simulink model "UAM_Flight_control"  (R2024b)
settings: Solver=FixedStepAuto  StartTime=0.0  StopTime=inf  RelTol=1e-3  EnableMultiTasking=on
undefined symbols (not defined in the file): CityMission, control, controlParams, ControlSampleTime, Cruise_a, DiscIntNeverNeededParam, Earth, FixedWingMission, flightState, FSState, FWControlParams, FWTrimSpeed, HoverMission, params, position, R_WAYPOINTTRANSITION, TransitionMission, uavParam, Vt, w_trim, WGS84, zGround
libraries: slpidlib x56, simulink x35, uavalgslib x8, robotcorelib x2, simulink_extras x2, mspfiltlib x1, aerolibtransform2 x1
(part 3 of 12)

== system UAM_Flight_control/GNC/Guidance/Auto ==
  note: Ground : 해발고도 기준, 착륙 지점 고도
  Pose : Inport
  Mission : Inport  Port=2  OutDataTypeStr=Bus: UAVPathManagerBus
  isModeDone : Inport  Port=3
  LandingStates : Inport  Port=4
  States : Inport  Port=5
  Ground : Inport  Port=6
  Action Port : ActionPort  ActionPortLabel=case [ Auto ]:
  Bus Creator : BusCreator  Inputs=6  OutDataTypeStr=Bus: GNCplan
  Bus Creator1 : BusCreator  Inputs=3  OutDataTypeStr=Bus: UAVPathManagerBus  NonVirtualBus=on
  Bus Selector : BusSelector  OutputSignals=mode
  Bus Selector1 : BusSelector  OutputSignals=target
  Compare To Constant : simulink/Logic and Bit Operations/Compare To Constant  relop===  const=1  OutDataTypeStr=boolean
  Compare To Constant1 : simulink/Logic and Bit Operations/Compare To Constant  relop=>=  const=3.0  OutDataTypeStr=boolean
  Constant : Constant  Value=0  OutDataTypeStr=uint8
  Constant1 : Constant  Value=[0,0,0]  OutDataTypeStr=double
  Constant2 : Constant  OutDataTypeStr=uint8
  Constant3 : Constant  Value=[0;0;0;0]
  Goto : Goto  Commented=on  GotoTag=landingState
  IC : InitialCondition
  Logical Operator : Logic  Operator=OR  Inputs=1  AllPortsSameDT=off  OutDataTypeStr=boolean
  Path Manager : uavalgslib/Path Manager  UAVType=multirotor  LoiterRadius=25  dataType=double  inputBusName='UAVPathManagerBus'  SimulateUsing=Code generation
  Reshape : Reshape  OutputDimensionality=Customize  OutputDimensions=[3 1]
  Selector : Selector  InputPortWidth=2  IndexOptions=Index vector (dialog)  Indices=1  OutputSizes=1
  Selector1 : Selector  InputPortWidth=2  IndexOptions=Index vector (dialog)  Indices=2  OutputSizes=1
  Switch : Switch  Criteria=u2 > Threshold  SaturateOnIntegerOverflow=off  InputSameDT=off
  GNCPlan : Outport  OutDataTypeStr=Bus: GNCplan
  wires:
  IC/1 -> Bus Creator/1  "mode"
  Ground/1 -> Bus Creator/6  "ground"
  Selector1/1 -> Bus Creator/3  "FromWP"
  States/1 -> Bus Selector1/1, Bus Creator/5  "states"
  Bus Creator/1 -> GNCPlan/1
  Selector/1 -> Bus Selector/1, Switch/3  "ToWP"
  Path Manager/1 -> Selector/1, Selector1/1
  Constant/1 -> Path Manager/4
  Constant1/1 -> Path Manager/5
  Pose/1 -> Bus Creator/4, Path Manager/1  "pose"
  LandingStates/1 -> Goto/1
  Compare To Constant/1 -> Path Manager/3
  isModeDone/1 -> Compare To Constant/1
  Bus Selector/1 -> IC/1  "<mode>"
  Mission/1 -> Path Manager/2
  Bus Selector1/1 -> Reshape/1, Compare To Constant1/1  "<target>"
  Compare To Constant1/1 -> Logical Operator/1
  Logical Operator/1 -> Switch/2
  Switch/1 -> Bus Creator/2  "ToWP"
  Constant2/1 -> Bus Creator1/1  "mode"
  Constant3/1 -> Bus Creator1/3  "params"
  Reshape/1 -> Bus Creator1/2  "position"
  Bus Creator1/1 -> Switch/1

== system UAM_Flight_control/GNC/Guidance/Emergency ==
  pose : Inport
  states : Inport  Port=2
  ground : Inport  Port=3
  Action Port : ActionPort  ActionPortLabel=case [ Emergecny ]:
  Bus Creator : BusCreator  Inputs=6  OutDataTypeStr=Bus: GNCplan
  Constant1 : Constant  Value=struct('mode', uint8(0), 'position', zeros(3,1), 'params', zeros(4,1))  OutDataTypeStr=Bus: UAVPathManagerBus
  Constant2 : Constant  Value=struct('mode', uint8(0), 'position', zeros(3,1), 'params', zeros(4,1))  OutDataTypeStr=Bus: UAVPathManagerBus
  Constant3 : Constant  Value=0  OutDataTypeStr=uint8
  GNCPlan : Outport  OutDataTypeStr=Bus: GNCplan
  wires:
  pose/1 -> Bus Creator/4  "pose"
  Bus Creator/1 -> GNCPlan/1
  Constant1/1 -> Bus Creator/2  "ToWP"
  Constant2/1 -> Bus Creator/3  "FromWP"
  ground/1 -> Bus Creator/6  "ground"
  states/1 -> Bus Creator/5  "states"
  Constant3/1 -> Bus Creator/1  "mode"

== system UAM_Flight_control/GNC/Guidance/Switch Case Action Subsystem ==
  pose : Inport
  states : Inport  Port=2
  ground : Inport  Port=3
  Action Port : ActionPort  ActionPortLabel=case [ Manual ]:
  Bus Creator : BusCreator  Inputs=6  OutDataTypeStr=Bus: GNCplan
  Constant1 : Constant  Value=struct('mode', uint8(0), 'position', zeros(3,1), 'params', zeros(4,1))  OutDataTypeStr=Bus: UAVPathManagerBus
  Constant2 : Constant  Value=struct('mode', uint8(0), 'position', zeros(3,1), 'params', zeros(4,1))  OutDataTypeStr=Bus: UAVPathManagerBus
  Constant3 : Constant  Value=0  OutDataTypeStr=uint8
  GNCPlan : Outport  OutDataTypeStr=Bus: GNCplan
  wires:
  Bus Creator/1 -> GNCPlan/1
  Constant3/1 -> Bus Creator/1  "mode"
  Constant2/1 -> Bus Creator/3  "FromWP"
  Constant1/1 -> Bus Creator/2  "ToWP"
  pose/1 -> Bus Creator/4  "pose"
  states/1 -> Bus Creator/5  "states"
  ground/1 -> Bus Creator/6  "ground"

== system UAM_Flight_control/GNC/Guidance/UAM POS ==
  UAMStates : Inport  OutDataTypeStr=Bus: StateBus
  Bus Creator : BusCreator  Inputs=5
  Bus Selector : BusSelector  OutputSignals=Xe,Ve
  Demux : Demux  Outputs=3
  Display : Display
  Selector : Selector  InputPortWidth=3  IndexOptions=Index vector (dialog)  Indices=[1]  OutputSizes=1
  Selector1 : Selector  InputPortWidth=3  IndexOptions=Index vector (dialog)  Indices=[2]  OutputSizes=1
  POS : Outport
  wires:
  UAMStates/1 -> Bus Selector/1
  Bus Selector/1 -> Demux/1  "<Xe>"
  Demux/1 -> Bus Creator/1  "x"
  Demux/2 -> Bus Creator/2  "y"
  Demux/3 -> Bus Creator/3  "z"
  Bus Selector/2 -> Selector/1, Selector1/1  "<Ve>"
  Selector/1 -> Bus Creator/4  "vx"
  Selector1/1 -> Bus Creator/5  "vy"
  Bus Creator/1 -> Display/1, POS/1

== system UAM_Flight_control/GNC/Guidance/UAM States ==
  UAMStates : Inport
  Bus Creator : BusCreator  Inputs=8
  Bus Selector : BusSelector  OutputSignals=Euler,pqr,Ve,Xe,course,RotorParameters,RC,target
  States : Outport
  wires:
  UAMStates/1 -> Bus Selector/1
  Bus Creator/1 -> States/1
  Bus Selector/1 -> Bus Creator/1  "<Euler>"
  Bus Selector/2 -> Bus Creator/2  "<pqr>"
  Bus Selector/3 -> Bus Creator/3  "<Ve>"
  Bus Selector/5 -> Bus Creator/5  "<course>"
  Bus Selector/4 -> Bus Creator/4  "<Xe>"
  Bus Selector/6 -> Bus Creator/6  "<RotorParameters>"
  Bus Selector/7 -> Bus Creator/7  "<RC>"
  Bus Selector/8 -> Bus Creator/8  "<target>"

== system UAM_Flight_control/GNC/Navigation/LLA2Local ==
  LLA : Inport
  ve : Inport  Port=2
  Enabled Subsystem : Subsystem  Commented=on  TreatAsAtomicUnit=on
  MATLAB Function : MATLAB Function  TreatAsAtomicUnit=on
  Xe : Outport
  wires:
  LLA/1 -> MATLAB Function/1(LLA)
  ve/1 -> MATLAB Function/2(arming)
  MATLAB Function/1(Xe) -> Xe/1

== system UAM_Flight_control/Sensor/Subsystem1/Subsystem ==
  Inport : Inport
  Gain2 : Gain  Gain=0.5
  Gyro_bias : Constant  Value=[-0.000114; -0.000246; -0.001536]
  MATLAB Function1 : MATLAB Function  TreatAsAtomicUnit=on
  MATLAB Function2 : MATLAB Function  TreatAsAtomicUnit=on
  Sum : Sum  Inputs=|+-
  Unit Delay : UnitDelay  InitialCondition=[1;0;0;0]  SampleTime=-1  HasFrameUpgradeWarning=on
  dt : Gain  Gain=0.005
  normalize : MATLAB Function  TreatAsAtomicUnit=on
  qn : Outport
  wires:
  Sum/1 -> Gain2/1
  MATLAB Function2/1(qout) -> normalize/1(q)
  normalize/1(qn) -> qn/1, Unit Delay/1
  Gyro_bias/1 -> Sum/2
  Unit Delay/1 -> MATLAB Function2/1(q)
  Gain2/1 -> dt/1
  Inport/1 -> Sum/1
  dt/1 -> MATLAB Function1/1(theta)
  MATLAB Function1/1(dq) -> MATLAB Function2/2(dq)

== system UAM_Flight_control/Controller/Auto1/Blend Scheduler/BTalpha ==
  States : Inport
  Bus Selector : BusSelector  OutputSignals=airspeed
  Constant : Constant  Value=65
  Gain : Gain  Gain=1/20
  Saturation : Saturate  UpperLimit=1  LowerLimit=0
  Subtract : Sum  Inputs=+-
  alpha : Outport
  wires:
  Constant/1 -> Subtract/1
  Subtract/1 -> Gain/1
  Gain/1 -> Saturation/1
  Saturation/1 -> alpha/1
  States/1 -> Bus Selector/1
  Bus Selector/1 -> Subtract/2  "<airspeed>"

== system UAM_Flight_control/Controller/Auto1/Blend Scheduler/FTalpha ==
  States : Inport
  1-a : Sum  Inputs=+-
  Bus Selector : BusSelector  OutputSignals=airspeed
  Constant3 : Constant  Value=35
  Constant5 : Constant  Value=Cruise_a
  Gain3 : Gain  Gain=1/10
  Saturation1 : Saturate  UpperLimit=10  LowerLimit=0
  Sum2 : Sum  Inputs=|+-
  alpha : Outport
  wires:
  1-a/1 -> alpha/1
  Bus Selector/1 -> Sum2/1  "<airspeed>"
  Gain3/1 -> 1-a/2
  Sum2/1 -> Saturation1/1
  Saturation1/1 -> Gain3/1
  Constant3/1 -> Sum2/2
  States/1 -> Bus Selector/1
  Constant5/1 -> 1-a/1

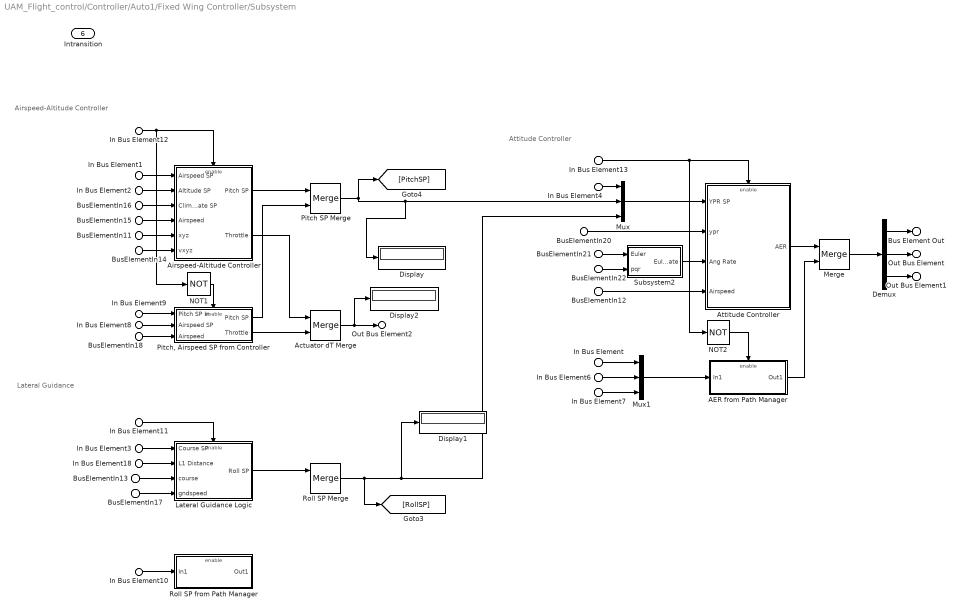
== system UAM_Flight_control/Controller/Auto1/Fixed Wing Controller/Subsystem ==
  note: Airspeed-Altitude Controller
  note: Lateral Guidance
  note: Attitude Controller
  BusElementIn11 : Inport  PortName=States  Element=Xe
  BusElementIn12 : Inport  PortName=States  Element=airspeed
  BusElementIn15 : Inport  PortName=States  Element=airspeed
  BusElementIn18 : Inport  PortName=States  Element=airspeed
  BusElementIn13 : Inport  PortName=States  Element=course
  BusElementIn16 : Inport  PortName=States  Element=course
  BusElementIn14 : Inport  PortName=States  Element=Ve_ground
  BusElementIn17 : Inport  PortName=States  Element=gndspeed
  BusElementIn20 : Inport  PortName=States  Element=YPR
  BusElementIn21 : Inport  PortName=States  Element=Euler
  BusElementIn22 : Inport  PortName=States  Element=pqr
  In Bus Element11 : Inport  Port=2  PortName=Control Mode  Element=lateralGuidance
  In Bus Element12 : Inport  Port=2  PortName=Control Mode  Element=airspeedAltitude
  In Bus Element13 : Inport  Port=2  PortName=Control Mode  Element=attitude
  In Bus Element1 : Inport  Port=3  PortName=AAC SP  Element=airspeed
  In Bus Element2 : Inport  Port=3  PortName=AAC SP  Element=altitude
  In Bus Element18 : Inport  Port=3  PortName=AAC SP  Element=L1
  In Bus Element3 : Inport  Port=3  PortName=AAC SP  Element=course
  In Bus Element4 : Inport  Port=4  PortName=FixedWingSP  Element=yaw
  In Bus Element9 : Inport  Port=4  PortName=FixedWingSP  Element=pitch
  In Bus Element10 : Inport  Port=4  PortName=FixedWingSP  Element=roll
  In Bus Element8 : Inport  Port=4  PortName=FixedWingSP  Element=airspeed
  In Bus Element : Inport  Port=5  PortName=AERT  Element=aileron
  In Bus Element6 : Inport  Port=5  PortName=AERT  Element=elevator
  In Bus Element7 : Inport  Port=5  PortName=AERT  Element=rudder
  Intransition : Inport  Port=6
  AER from Path Manager : Subsystem  TreatAsAtomicUnit=on
  Actuator dT Merge : Merge
  Airspeed-Altitude Controller : Subsystem
  Attitude Controller : Subsystem
  Demux : Demux  Outputs=3
  Display : Display
  Display1 : Display
  Display2 : Display
  Lateral Guidance Logic : Subsystem
  Merge : Merge
  Mux : Mux  Inputs=3
  Mux1 : Mux  Inputs=3
  NOT1 : Logic  Operator=NOT  IconShape=distinctive  AllPortsSameDT=off  OutDataTypeStr=boolean
  NOT2 : Logic  Operator=NOT  IconShape=distinctive  AllPortsSameDT=off  OutDataTypeStr=boolean
  Pitch SP Merge : Merge
  "Pitch, Airspeed SP from Controller" : Subsystem  TreatAsAtomicUnit=on
  Roll SP Merge : Merge
  Roll SP from Path Manager : Subsystem  TreatAsAtomicUnit=on
  Subsystem2 : Subsystem
  Bus Element Out : Outport  PortName=Actuator  Element=dA
  Out Bus Element : Outport  PortName=Actuator  Element=dE
  Out Bus Element1 : Outport  PortName=Actuator  Element=dR
  Out Bus Element2 : Outport  PortName=Actuator  Element=dT
  wires:
  In Bus Element4/1 -> Mux/1
  Roll SP Merge/1 -> [RollSP], Display1/1, Mux/3
  BusElementIn18/1 -> "Pitch, Airspeed SP from Controller"/3(Airspeed)
  In Bus Element12/1 -> Airspeed-Altitude Controller/Enable, NOT1/1
  In Bus Element3/1 -> Lateral Guidance Logic/1(Course SP)
  Mux1/1 -> AER from Path Manager/1(In1)
  In Bus Element11/1 -> Lateral Guidance Logic/Enable
  Lateral Guidance Logic/1(Roll SP) -> Roll SP Merge/1
  In Bus Element7/1 -> Mux1/3
  Demux/2 -> Out Bus Element/1
  Demux/1 -> Bus Element Out/1
  In Bus Element9/1 -> "Pitch, Airspeed SP from Controller"/1(Pitch SP In)
  Merge/1 -> Demux/1
  In Bus Element18/1 -> Lateral Guidance Logic/2(L1 Distance)
  In Bus Element13/1 -> NOT2/1, Attitude Controller/Enable
  "Pitch, Airspeed SP from Controller"/1(Pitch SP) -> Pitch SP Merge/2
  BusElementIn14/1 -> Airspeed-Altitude Controller/6(vxyz)
  Pitch SP Merge/1 -> Display/1, Mux/2, [PitchSP]
  BusElementIn15/1 -> Airspeed-Altitude Controller/4(Airspeed)
  In Bus Element8/1 -> "Pitch, Airspeed SP from Controller"/2(Airspeed SP)
  BusElementIn13/1 -> Lateral Guidance Logic/3(course)
  Airspeed-Altitude Controller/2(Throttle) -> Actuator dT Merge/1
  BusElementIn16/1 -> Airspeed-Altitude Controller/3(Climb Rate SP)
  In Bus Element1/1 -> Airspeed-Altitude Controller/1(Airspeed SP)
  BusElementIn11/1 -> Airspeed-Altitude Controller/5(xyz)
  BusElementIn12/1 -> Attitude Controller/4(Airspeed)
  In Bus Element2/1 -> Airspeed-Altitude Controller/2(Altitude SP)
  BusElementIn20/1 -> Attitude Controller/2(ypr)
  Mux/1 -> Attitude Controller/1(YPR SP)
  Demux/3 -> Out Bus Element1/1
  BusElementIn21/1 -> Subsystem2/1(Euler)
  Subsystem2/1(Euler Rate) -> Attitude Controller/3(Ang Rate)
  "Pitch, Airspeed SP from Controller"/2(Throttle) -> Actuator dT Merge/2
  Airspeed-Altitude Controller/1(Pitch SP) -> Pitch SP Merge/1
  Attitude Controller/1(AER) -> Merge/1
  AER from Path Manager/1(Out1) -> Merge/2
  In Bus Element/1 -> Mux1/1
  In Bus Element10/1 -> Roll SP from Path Manager/1(In1)
  In Bus Element6/1 -> Mux1/2
  NOT2/1 -> AER from Path Manager/Enable
  BusElementIn22/1 -> Subsystem2/2(pqr)
  Actuator dT Merge/1 -> Display2/1, Out Bus Element2/1
  BusElementIn17/1 -> Lateral Guidance Logic/4(gndspeed)
  NOT1/1 -> "Pitch, Airspeed SP from Controller"/Enable

== system UAM_Flight_control/Controller/Auto1/Multicopter Controller/Attitude & Altitude controller ==
  Ref Attitude : Inport
  States : Inport  Port=2
  Z ref : Inport  Port=3
  InTransition : Inport  Port=4
  CtrlMode : Inport  Port=5
  FlightMode : Inport  Port=6
  Altitude Control : Subsystem
  Bus Selector : BusSelector  OutputSignals=RC
  Compare To Constant : simulink/Logic and Bit Operations/Compare To Constant  relop=>  const=1700  OutDataTypeStr=boolean
  Derivative Gain : Subsystem  VariantControl=AttitudeControl==1
  Selector : Selector  InputPortWidth=10  IndexOptions=Index vector (dialog)  Indices=7  OutputSizes=1
  Roll torque cmd : Outport
  Pitch torque Cmd : Outport  Port=2
  Yaw torque Cmd : Outport  Port=3
  commanded thrust : Outport  Port=4
  wires:
  Altitude Control/1(commanded thrust) -> commanded thrust/1
  Derivative Gain/1(Roll torque cmd) -> Roll torque cmd/1
  InTransition/1 -> Altitude Control/3(InTransition)
  Derivative Gain/2(Pitch torque Cmd) -> Pitch torque Cmd/1
  States/1 -> Derivative Gain/2(States), Bus Selector/1, Altitude Control/1(States)
  Derivative Gain/3(Yaw torque Cmd) -> Yaw torque Cmd/1
  Z ref/1 -> Altitude Control/2(Z ref)
  FlightMode/1 -> Altitude Control/4(FlightMode)
  Ref Attitude/1 -> Derivative Gain/1(Ref Attitude)
  Selector/1 -> Compare To Constant/1
  Bus Selector/1 -> Selector/1  "<RC>"
  Compare To Constant/1 -> Altitude Control/Enable
  CtrlMode/1 -> Derivative Gain/3(CtrlMode), Altitude Control/5(CtrlMode)

== system UAM_Flight_control/Controller/Auto1/Multicopter Controller/Horizontal Position Control ==
  note: Forward Motion is controlled using Tilt.
      | Lateral Motion occurs using roll.
  XRef : Inport
  YRef : Inport  Port=2
  States : Inport  Port=3
  Enable : EnablePort  ShowOutputPort=on
  Signal Conversion : SignalConversion  OverrideOpt=off
  Signal Conversion1 : SignalConversion  OverrideOpt=off
  XY Controller : Subsystem
  Roll Cmd : Outport
  Pitch Cmd : Outport  Port=2
  wires:
  XRef/1 -> XY Controller/1(X_ref)
  YRef/1 -> XY Controller/2(Y_ref)
  States/1 -> XY Controller/3(States)
  XY Controller/1(Forward cmd) -> Signal Conversion/1
  XY Controller/2(Sideward Cmd) -> Signal Conversion1/1
  Signal Conversion/1 -> Pitch Cmd/1
  Signal Conversion1/1 -> Roll Cmd/1
  Enable/1 -> XY Controller/Enable

== system UAM_Flight_control/Controller/Auto1/Multicopter Controller/Organize Inputs ==
  forward command : Inport
  commanded phi torque : Inport  Port=2
  commanded theta torque : Inport  Port=3
  commanded psi torque : Inport  Port=4
  commanded thrust : Inport  Port=5
  Out Bus Element : Outport  PortName=MixerCommands  Element=w_phi
  Out Bus Element1 : Outport  PortName=MixerCommands  Element=w_theta
  Out Bus Element2 : Outport  PortName=MixerCommands  Element=w_psi
  Out Bus Element3 : Outport  PortName=MixerCommands  Element=w_z
  Out Bus Element4 : Outport  PortName=MixerCommands  Element=l_x
  wires:
  forward command/1 -> Out Bus Element4/1
  commanded phi torque/1 -> Out Bus Element/1  "phi"
  commanded theta torque/1 -> Out Bus Element1/1
  commanded psi torque/1 -> Out Bus Element2/1
  commanded thrust/1 -> Out Bus Element3/1

== system UAM_Flight_control/Controller/Auto1/Multicopter Controller/transition controller ==
  Enable : EnablePort
  Constant : Constant  Value=0
  Constant1 : Constant  Value=0
  Rollcmd : Outport
  Pitchcmd : Outport  Port=2
  wires:
  Constant/1 -> Rollcmd/1
  Constant1/1 -> Pitchcmd/1

== system UAM_Flight_control/Controller/Auto1/Scheduler/FixedWingScheduler ==
  note: C opyright 2024 The MathWorks, Inc.
  note: Fixed Wing Control Mixer
  FlightState : Inport
  FixedWingActuators : Inport  Port=2  OutDataTypeStr=Bus: FixedWingCtrlBus
  Merge : Merge  Inputs=4
  Switch Case : SwitchCase  CaseConditions={flightState.Hover, flightState.Transition, flightState.FixedWing,flightState.BackTransition}  ShowDefaultCase=off
  Switch Case Action Subsystem : Subsystem  TreatAsAtomicUnit=on
  Switch Case Action Subsystem1 : Subsystem  TreatAsAtomicUnit=on
  Switch Case Action Subsystem2 : Subsystem  TreatAsAtomicUnit=on
  Switch Case Action Subsystem3 : Subsystem  TreatAsAtomicUnit=on
  ActuatorControls : Outport
  wires:
  FlightState/1 -> Switch Case/1
  FixedWingActuators/1 -> Switch Case Action Subsystem2/1(FixedWingActuators), Switch Case Action Subsystem1/1(FixedWingActuators)
  Switch Case/3 -> Switch Case Action Subsystem2/Action
  Switch Case/2 -> Switch Case Action Subsystem1/Action
  Switch Case Action Subsystem3/1(FixedWingControls) -> Merge/4
  Merge/1 -> ActuatorControls/1
  Switch Case Action Subsystem1/1(FixedWingControls) -> Merge/2
  Switch Case/4 -> Switch Case Action Subsystem3/Action
  Switch Case Action Subsystem/1(FixedWingControls) -> Merge/1
  Switch Case/1 -> Switch Case Action Subsystem/Action
  Switch Case Action Subsystem2/1(FixedWingControls) -> Merge/3

== system UAM_Flight_control/Controller/Auto1/Scheduler/Subsystem ==
  note: C opyright 2024 The MathWorks, Inc.
  note: Multicopter Control Mixer
  FlightState : Inport
  FixedWingActuators : Inport  Port=2
  CtrlMode : Inport  Port=3
  MotorCommands : Inport  Port=4
  Actuator To Voltage : Subsystem
  Merge : Merge  Inputs=4
  Switch Case : SwitchCase  CaseConditions={flightState.Hover, flightState.Transition, flightState.FixedWing,flightState.BackTransition}  ShowDefaultCase=off
  Switch Case Action Subsystem : Subsystem  TreatAsAtomicUnit=on
  Switch Case Action Subsystem1 : Subsystem  TreatAsAtomicUnit=on
  Switch Case Action Subsystem2 : Subsystem  TreatAsAtomicUnit=on
  Switch Case Action Subsystem3 : Subsystem  TreatAsAtomicUnit=on
  ActuatorControls : Outport  OutDataTypeStr=Bus: FCCData
  wires:
  Switch Case/4 -> Switch Case Action Subsystem3/Action
  MotorCommands/1 -> Switch Case Action Subsystem3/1(MixerCommands), Switch Case Action Subsystem/1(MixerCommands), Switch Case Action Subsystem1/1(MixerCommands)
  FlightState/1 -> Switch Case/1
  Switch Case Action Subsystem3/1(Actuator) -> Merge/4
  FixedWingActuators/1 -> Switch Case Action Subsystem2/1(FixedWingCtrlBus)
  Switch Case/3 -> Switch Case Action Subsystem2/Action
  Switch Case/2 -> Switch Case Action Subsystem1/Action
  Switch Case Action Subsystem1/1(Actuator) -> Merge/2
  Switch Case/1 -> Switch Case Action Subsystem/Action
  Switch Case Action Subsystem2/1(Actuator) -> Merge/3
  Switch Case Action Subsystem/1(Actuator) -> Merge/1
  Merge/1 -> Actuator To Voltage/2(Motor Commands)
  Actuator To Voltage/1(Actuator) -> ActuatorControls/1
  CtrlMode/1 -> Actuator To Voltage/1(CtrlMode)

== system UAM_Flight_control/Controller/Emergency/FixedWing Controller/Subsystem ==
  note: Attitude Controller
  BusElementIn4 : Inport  PortName=States  Element=pqr
  BusElementIn5 : Inport  PortName=States  Element=Euler
  BusElementIn6 : Inport  PortName=States  Element=YPR
  BusElementIn7 : Inport  PortName=States  Element=airspeed
  In Bus Element13 : Inport  Port=2  PortName=Control Mode  Element=attitude
  RC : Inport  Port=3
  Attitude Controller : Subsystem
  Demux : Demux  Outputs=3
  Demux1 : Demux  Outputs=10
  Mux : Mux  Inputs=3
  Subsystem2 : Subsystem
  Terminator{1..6} (6 alike) : Terminator
  normalization : Subsystem
  normalization1 : Subsystem
  normalization2 : Subsystem
  Bus Element Out : Outport  PortName=Actuator  Element=dA
  Out Bus Element : Outport  PortName=Actuator  Element=dE
  Out Bus Element1 : Outport  PortName=Actuator  Element=dR
  Out Bus Element2 : Outport  PortName=Actuator  Element=dT
  wires:
  Demux/2 -> Out Bus Element/1
  Demux/1 -> Bus Element Out/1
  In Bus Element13/1 -> Attitude Controller/Enable
  BusElementIn7/1 -> Attitude Controller/4(Airspeed)
  BusElementIn6/1 -> Attitude Controller/2(ypr)
  Mux/1 -> Attitude Controller/1(YPR SP)
  Demux/3 -> Out Bus Element1/1
  BusElementIn5/1 -> Subsystem2/1(Euler)
  Subsystem2/1(Euler Rate) -> Attitude Controller/3(Ang Rate)
  Attitude Controller/1(AER) -> Demux/1
  BusElementIn4/1 -> Subsystem2/2(pqr)
  RC/1 -> Demux1/1
  Demux1/1 -> normalization1/1(In1)  "roll"
  Demux1/2 -> normalization2/1(In1)  "pitch"
  Demux1/3 -> Out Bus Element2/1  "throttle"
  Demux1/4 -> normalization/1(In1)  "yaw"
  Demux1/5 -> Terminator1/1
  normalization/1(Out1) -> Mux/1
  normalization1/1(Out1) -> Mux/2
  normalization2/1(Out1) -> Mux/3
  Demux1/6 -> Terminator2/1
  Demux1/7 -> Terminator3/1
  Demux1/8 -> Terminator4/1
  Demux1/9 -> Terminator5/1
  Demux1/10 -> Terminator6/1

== system UAM_Flight_control/Controller/Emergency/Scheduler/FixedWingScheduler ==
  note: C opyright 2024 The MathWorks, Inc.
  note: Fixed Wing Control Mixer
  FlightState : Inport
  FixedWingActuators : Inport  Port=2  OutDataTypeStr=Bus: FixedWingCtrlBus
  TransitionDone : Inport  Port=3
  Merge : Merge  Inputs=4
  Switch Case : SwitchCase  CaseConditions={flightState.Hover, flightState.Transition, flightState.FixedWing,flightState.BackTransition}  ShowDefaultCase=off
  Switch Case Action Subsystem : Subsystem  TreatAsAtomicUnit=on
  Switch Case Action Subsystem1 : Subsystem  TreatAsAtomicUnit=on
  Switch Case Action Subsystem2 : Subsystem  TreatAsAtomicUnit=on
  Switch Case Action Subsystem3 : Subsystem  TreatAsAtomicUnit=on
  ActuatorControls : Outport  OutDataTypeStr=Bus: FixedWingCtrlBus
  wires:
  FlightState/1 -> Switch Case/1
  FixedWingActuators/1 -> Switch Case Action Subsystem2/1(FixedWingActuators), Switch Case Action Subsystem1/1(FixedWingActuators)
  Switch Case/3 -> Switch Case Action Subsystem2/Action
  Switch Case/2 -> Switch Case Action Subsystem1/Action
  TransitionDone/1 -> Switch Case Action Subsystem1/2(TransitionDone)
  Switch Case Action Subsystem3/1(FixedWingControls) -> Merge/4
  Merge/1 -> ActuatorControls/1
  Switch Case Action Subsystem1/1(FixedWingControls) -> Merge/2
  Switch Case/4 -> Switch Case Action Subsystem3/Action
  Switch Case Action Subsystem/1(FixedWingControls) -> Merge/1
  Switch Case/1 -> Switch Case Action Subsystem/Action
  Switch Case Action Subsystem2/1(FixedWingControls) -> Merge/3

== system UAM_Flight_control/Controller/Emergency/Scheduler/Subsystem ==
  note: C opyright 2024 The MathWorks, Inc.
  note: Multicopter Control Mixer
  FlightState : Inport
  FixedWingActuators : Inport  Port=2
  MotorCommands : Inport  Port=3
  BlendingSchedule : Inport  Port=4
  TransitionDone : Inport  Port=5
  BackTransitionDone : Inport  Port=6
  Actuator To Voltage : Subsystem
  Merge : Merge  Inputs=4
  Switch Case : SwitchCase  CaseConditions={flightState.Hover, flightState.Transition, flightState.FixedWing,flightState.BackTransition}  ShowDefaultCase=off
  Switch Case Action Subsystem : Subsystem  TreatAsAtomicUnit=on
  Switch Case Action Subsystem1 : Subsystem  TreatAsAtomicUnit=on
  Switch Case Action Subsystem2 : Subsystem  TreatAsAtomicUnit=on
  Switch Case Action Subsystem3 : Subsystem  TreatAsAtomicUnit=on
  ActuatorControls : Outport  OutDataTypeStr=Bus: FCCData
  wires:
  Switch Case/4 -> Switch Case Action Subsystem3/Action
  MotorCommands/1 -> Switch Case Action Subsystem3/2(MixerCommands), Switch Case Action Subsystem/1(MixerCommands), Switch Case Action Subsystem1/2(MixerCommands)
  FlightState/1 -> Switch Case/1
  Switch Case Action Subsystem/1(Actuator) -> Merge/1
  Switch Case Action Subsystem3/1(Actuator) -> Merge/4
  FixedWingActuators/1 -> Switch Case Action Subsystem2/1(FixedWingCtrlBus), Switch Case Action Subsystem1/3(FixedWing)
  Switch Case/3 -> Switch Case Action Subsystem2/Action
  TransitionDone/1 -> Switch Case Action Subsystem1/4(TransitionDone)
  Switch Case/2 -> Switch Case Action Subsystem1/Action
  Switch Case Action Subsystem1/1(Actuator) -> Merge/2
  BlendingSchedule/1 -> Switch Case Action Subsystem1/1(BlendingSchedule), Switch Case Action Subsystem3/1(BlendingSchedule)
  Switch Case/1 -> Switch Case Action Subsystem/Action
  BackTransitionDone/1 -> Switch Case Action Subsystem3/3(BackTransitionDone)
  Switch Case Action Subsystem2/1(Actuator) -> Merge/3
  Actuator To Voltage/1(Actuator) -> ActuatorControls/1
  Merge/1 -> Actuator To Voltage/1(Motor Commands)

== system UAM_Flight_control/Controller/Emergency/multicopter Controller/Attitude & Altitude controller ==
  Ref Attitude : Inport
  States : Inport  Port=2
  Bias : Bias  Bias=-1500  SaturateOnIntegerOverflow=off
  Bus Selector : BusSelector  OutputSignals=RC
  Derivative Gain : Subsystem  VariantControl=AttitudeControl==1
  Display : Display
  Gain : Gain  Gain=1/500
  Selector : Selector  InputPortWidth=10  IndexOptions=Index vector (dialog)  Indices=3  OutputSizes=1
  Roll torque cmd : Outport
  Pitch torque Cmd : Outport  Port=2
  Yaw torque Cmd : Outport  Port=3
  commanded thrust : Outport  Port=4
  wires:
  Derivative Gain/1(Roll torque cmd) -> Roll torque cmd/1
  Derivative Gain/2(Pitch torque Cmd) -> Pitch torque Cmd/1
  States/1 -> Bus Selector/1, Derivative Gain/2(States)
  Derivative Gain/3(Yaw torque Cmd) -> Yaw torque Cmd/1
  Ref Attitude/1 -> Derivative Gain/1(Ref Attitude)
  Bus Selector/1 -> Selector/1  "<RC>"
  Selector/1 -> Bias/1
  Bias/1 -> Gain/1
  Gain/1 -> Display/1, commanded thrust/1

== system UAM_Flight_control/Controller/Emergency/multicopter Controller/Organize Inputs ==
  forward command : Inport
  commanded phi torque : Inport  Port=2
  commanded theta torque : Inport  Port=3
  commanded psi torque : Inport  Port=4
  commanded thrust : Inport  Port=5
  Display{,1..3} (4 alike) : Display
  Out Bus Element : Outport  PortName=MixerCommands  Element=w_phi
  Out Bus Element1 : Outport  PortName=MixerCommands  Element=w_theta
  Out Bus Element2 : Outport  PortName=MixerCommands  Element=w_psi
  Out Bus Element3 : Outport  PortName=MixerCommands  Element=w_z
  Out Bus Element4 : Outport  PortName=MixerCommands  Element=l_x
  wires:
  commanded theta torque/1 -> Display2/1, Out Bus Element1/1  "theta"
  commanded psi torque/1 -> Display1/1, Out Bus Element2/1
  commanded thrust/1 -> Display/1, Out Bus Element3/1
  forward command/1 -> Out Bus Element4/1
  commanded phi torque/1 -> Display3/1, Out Bus Element/1  "phi"

== system UAM_Flight_control/Controller/Manual/FixedWing Controller/Subsystem ==
  BusElementIn4 : Inport  PortName=States  Element=pqr
  BusElementIn5 : Inport  PortName=States  Element=airspeed
  BusElementIn6 : Inport  PortName=States  Element=Euler
  BusElementIn7 : Inport  PortName=States  Element=YPR
  In Bus Element13 : Inport  Port=2  PortName=Control Mode  Element=attitude
  RC : Inport  Port=3
  Attitude Controller : Subsystem
  Demux : Demux  Outputs=3
  Demux1 : Demux  Outputs=10
  Mux : Mux  Inputs=3
  Subsystem2 : Subsystem
  Terminator{1..6} (6 alike) : Terminator
  normalization : Subsystem
  normalization1 : Subsystem
  normalization2 : Subsystem
  Bus Element Out : Outport  PortName=Actuator  Element=dA
  Out Bus Element : Outport  PortName=Actuator  Element=dE
  Out Bus Element1 : Outport  PortName=Actuator  Element=dR
  Out Bus Element2 : Outport  PortName=Actuator  Element=dT
  wires:
  Demux/2 -> Out Bus Element/1
  Demux/1 -> Bus Element Out/1
  In Bus Element13/1 -> Attitude Controller/Enable
  BusElementIn5/1 -> Attitude Controller/4(Airspeed)
  BusElementIn7/1 -> Attitude Controller/2(ypr)
  Mux/1 -> Attitude Controller/1(YPR SP)
  Demux/3 -> Out Bus Element1/1
  BusElementIn6/1 -> Subsystem2/1(Euler)
  Subsystem2/1(Euler Rate) -> Attitude Controller/3(Ang Rate)
  Attitude Controller/1(AER) -> Demux/1
  BusElementIn4/1 -> Subsystem2/2(pqr)
  RC/1 -> Demux1/1
  Demux1/1 -> normalization1/1(In1)  "roll"
  Demux1/2 -> normalization2/1(In1)  "pitch"
  Demux1/3 -> Out Bus Element2/1  "throttle"
  Demux1/4 -> normalization/1(In1)  "yaw"
  Demux1/5 -> Terminator1/1
  normalization/1(Out1) -> Mux/1
  normalization1/1(Out1) -> Mux/2
  normalization2/1(Out1) -> Mux/3
  Demux1/6 -> Terminator2/1
  Demux1/7 -> Terminator3/1
  Demux1/10 -> Terminator6/1
  Demux1/9 -> Terminator5/1
  Demux1/8 -> Terminator4/1

== system UAM_Flight_control/Controller/Manual/Scheduler/FixedWingScheduler ==
  note: C opyright 2024 The MathWorks, Inc.
  note: Fixed Wing Control Mixer
  FlightState : Inport
  FixedWingActuators : Inport  Port=2  OutDataTypeStr=Bus: FixedWingCtrlBus
  TransitionDone : Inport  Port=3
  Merge : Merge  Inputs=4
  Switch Case : SwitchCase  CaseConditions={flightState.Hover, flightState.Transition, flightState.FixedWing,flightState.BackTransition}  ShowDefaultCase=off
  Switch Case Action Subsystem : Subsystem  TreatAsAtomicUnit=on
  Switch Case Action Subsystem1 : Subsystem  TreatAsAtomicUnit=on
  Switch Case Action Subsystem2 : Subsystem  TreatAsAtomicUnit=on
  Switch Case Action Subsystem3 : Subsystem  TreatAsAtomicUnit=on
  ActuatorControls : Outport  OutDataTypeStr=Bus: FixedWingCtrlBus
  wires:
  FlightState/1 -> Switch Case/1
  FixedWingActuators/1 -> Switch Case Action Subsystem2/1(FixedWingActuators), Switch Case Action Subsystem1/1(FixedWingActuators)
  Switch Case/3 -> Switch Case Action Subsystem2/Action
  Switch Case/2 -> Switch Case Action Subsystem1/Action
  TransitionDone/1 -> Switch Case Action Subsystem1/2(TransitionDone)
  Switch Case Action Subsystem3/1(FixedWingControls) -> Merge/4
  Merge/1 -> ActuatorControls/1
  Switch Case Action Subsystem1/1(FixedWingControls) -> Merge/2
  Switch Case/4 -> Switch Case Action Subsystem3/Action
  Switch Case Action Subsystem/1(FixedWingControls) -> Merge/1
  Switch Case/1 -> Switch Case Action Subsystem/Action
  Switch Case Action Subsystem2/1(FixedWingControls) -> Merge/3

== system UAM_Flight_control/Controller/Manual/Scheduler/Subsystem ==
  note: C opyright 2024 The MathWorks, Inc.
  note: Multicopter Control Mixer
  FlightState : Inport
  FixedWingActuators : Inport  Port=2
  MotorCommands : Inport  Port=3
  BlendingSchedule : Inport  Port=4
  TransitionDone : Inport  Port=5
  BackTransitionDone : Inport  Port=6
  Actuator To Voltage : Subsystem
  Switch Case : SwitchCase  CaseConditions={flightState.Hover, flightState.Transition, flightState.FixedWing,flightState.BackTransition}  ShowDefaultCase=off
  Switch Case Action Subsystem : Subsystem  TreatAsAtomicUnit=on
  Switch Case Action Subsystem1 : Subsystem  TreatAsAtomicUnit=on
  Switch Case Action Subsystem2 : Subsystem  TreatAsAtomicUnit=on
  Switch Case Action Subsystem3 : Subsystem  TreatAsAtomicUnit=on
  ActuatorControls : Outport  OutDataTypeStr=Bus: FCCData
  wires:
  Switch Case/4 -> Switch Case Action Subsystem3/Action
  MotorCommands/1 -> Switch Case Action Subsystem3/2(MixerCommands), Switch Case Action Subsystem1/2(MixerCommands), Switch Case Action Subsystem/1(MixerCommands)
  FlightState/1 -> Switch Case/1
  FixedWingActuators/1 -> Switch Case Action Subsystem1/3(FixedWing), Switch Case Action Subsystem2/1(FixedWingCtrlBus)
  Switch Case/3 -> Switch Case Action Subsystem2/Action
  TransitionDone/1 -> Switch Case Action Subsystem1/4(TransitionDone)
  Switch Case/2 -> Switch Case Action Subsystem1/Action
  BlendingSchedule/1 -> Switch Case Action Subsystem3/1(BlendingSchedule), Switch Case Action Subsystem1/1(BlendingSchedule)
  Switch Case/1 -> Switch Case Action Subsystem/Action
  BackTransitionDone/1 -> Switch Case Action Subsystem3/3(BackTransitionDone)
  Actuator To Voltage/1(Actuator) -> ActuatorControls/1
  Switch Case Action Subsystem/1(Actuator) -> Actuator To Voltage/1(Motor Commands)

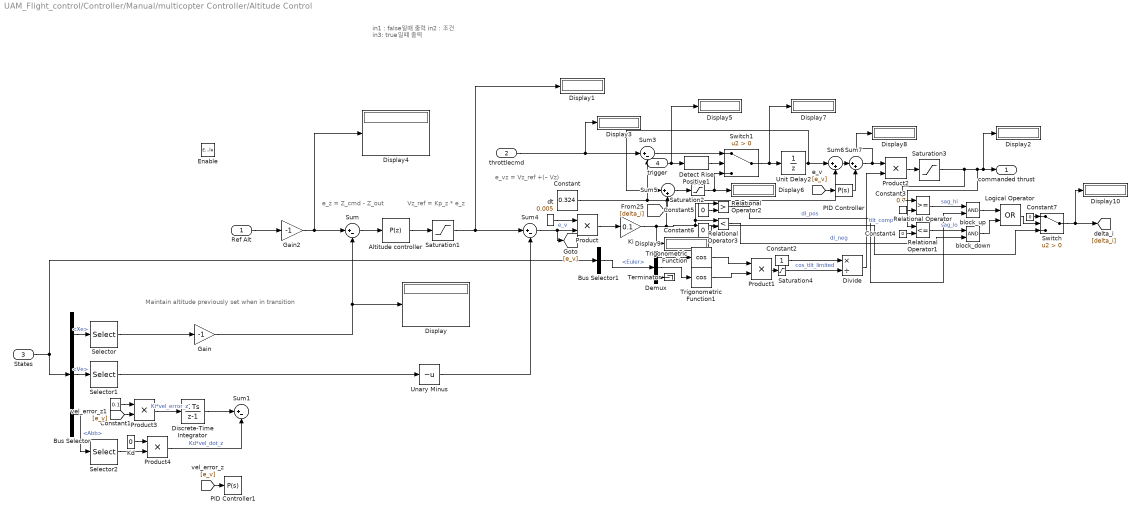
== system UAM_Flight_control/Controller/Manual/multicopter Controller/Altitude Control ==
  note: e_vz = Vz_ref +(– Vz)
  note: Vz_ref = Kp_z * e_z
  note: e_z = Z_cmd - Z_out
  note: in1 : false일때 출력
      | in2 : 조건
      | in3: true일떄 출력
  note: Maintain altitude previously set when in transition
  Ref Alt : Inport
  throttlecmd : Inport  Port=2
  States : Inport  Port=3
  trigger : Inport  Port=4
  Enable : EnablePort
  Altitude controller : slpidlib/PID Controller  Controller=P  Form=Parallel  TimeDomain=Discrete-time  UseExternalTs=off  SampleTime=-1  IntegratorMethod=Forward Euler  FilterMethod=Forward Euler  ControllerParametersSource=internal  P=controlParams.P_Z  I=controlParams.I_Z  UseKiTs=off  D=controlParams.D_Z  UseExternalDerivativeSource=off  N=controlParams.N_Z  UseFilter=on  TunerSelectOption=Transfer Function Based (PID Tuner App)  InitialConditionSource=internal  InitialConditionForIntegrator=0  InitialConditionForFilter=0  DifferentiatorICPrevScaledInput=0  ExternalReset=none  TrackingMode=off  Kt=1  LimitOutput=off  SatLimitsSource=internal  UpperSaturationLimit=inf  LowerSaturationLimit=-inf  LinearizeAsGain=on  AntiWindupMode=none  Kb=1  LimitIntegrator=off  UpperIntegratorSaturationLimit=inf  LowerIntegratorSaturationLimit=-inf  POutMin=[]  POutMax=[]  IOutMin=[]  IOutMax=[]  DOutMin=[]  DOutMax=[]  NOutMin=[]  NOutMax=[]  SumOutMin=[]  SumOutMax=[]  SaturationOutMin=[]  SaturationOutMax=[]  PParamMin=[]  PParamMax=[]  IParamMin=[]  IParamMax=[]  DParamMin=[]  DParamMax=[]  NParamMin=[]  NParamMax=[]  KbParamMin=[]  KbParamMax=[]  KtParamMin=[]  KtParamMax=[]  KbOutMin=[]  KbOutMax=[]  KtOutMin=[]  KtOutMax=[]  IntegratorOutMin=[]  IntegratorOutMax=[]  FilterOutMin=[]  FilterOutMax=[]  SumI1OutMin=[]  SumI1OutMax=[]  SumI2OutMin=[]  SumI2OutMax=[]  SumI3OutMin=[]  SumI3OutMax=[]  SumI4OutMin=[]  SumI4OutMax=[]  SumDOutMin=[]  SumDOutMax=[]  DifferentiatorOutMin=[]  DifferentiatorOutMax=[]  FilterDiffOutCoefMin=[]  FilterDiffOutCoefMax=[]  ReciprocalOutMin=[]  ReciprocalOutMax=[]  SumDenOutMin=[]  SumDenOutMax=[]  SumNumOutMin=[]  SumNumOutMax=[]  DivideOutMin=[]  DivideOutMax=[]  UdiffTsProdOutMin=[]  UdiffTsProdOutMax=[]  NTsProdOutMin=[]  NTsProdOutMax=[]  UintegralTsProdOutMin=[]  UintegralTsProdOutMax=[]  UngainTsProdOutMin=[]  UngainTsProdOutMax=[]  ClampingZeroOutDataTypeStr=Inherit: Inherit via back propagation  ClampingZeroOutMin=[]  ClampingZeroOutMax=[]  FilterDenConstantOutDataTypeStr=Inherit: Inherit via back propagation  FilterDenConstantOutMin=[]  FilterDenConstantOutMax=[]  PCopyOutDataTypeStr=Inherit: Inherit via back propagation  PCopyOutMin=[]  PCopyOutMax=[]  NCopyOutDataTypeStr=Inherit: Inherit via back propagation  NCopyOutMin=[]  NCopyOutMax=[]  IntegratorContinuousStateAttributes=''  IntegratorStateMustResolveToSignalObject=off  IntegratorRTWStateStorageClass=Auto  FilterContinuousStateAttributes=''  FilterStateMustResolveToSignalObject=off  FilterRTWStateStorageClass=Auto  ParallelPVariant=InternalParameters  IdealPVariant=Disabled  IVariant=Disabled  DVariant=Disabled  IntegratorVariant=Disabled  SatVariant=Disabled  AWVariant=Disabled  PCopyVariant=Disabled  TRVariant=Disabled  FdbkBlocksVariant=Forward  IdealPFdbkVariant=Disabled  SatFdbkVariant=Disabled  DerivativeFilterVariant=Disabled  NVariant=Disabled  NCopyVariant=Disabled_SignalSpec  FilterICVariant=Disabled  IntegratorICVariant=Disabled  ExternalResetVariant=Disabled  TRSumVariant=Passthrough  SumFdbkVariant=Disabled  SumVariant=Passthrough_P  TsampFilterVariant=InternalTs  TsampNgainVariant=Passthrough  TsampIntegralVariant=Disabled_SignalSpec  ExternalSaturationOutDataTypeStr=Inherit: Same as second input  DerivativeSourceVariant=Disabled  PreIntVariant=InternalPreInt
  Bus Selector : BusSelector  OutputSignals=Xe,Ve,Abb
  Bus Selector1 : BusSelector  OutputSignals=Euler
  Constant : Constant  Value=0.324
  Constant1 : Constant  Value=0.1
  Constant2 : Constant
  Constant3 : Constant  Value=0.7
  Constant{4..7} (4 alike) : Constant  Value=0
  Demux : Demux  Outputs=3
  Detect Rise Positive1 : simulink/Logic and Bit Operations/Detect Rise Positive  vinit=0  OutDataTypeStr=boolean
  Discrete-Time Integrator : DiscreteIntegrator  SampleTime=0.005  LimitOutput=on  UpperSaturationLimit=9.80665  LowerSaturationLimit=-9.80665  ICPrevOutput=DiscIntNeverNeededParam  ICPrevScaledInput=DiscIntNeverNeededParam
  Display{,1..10} (11 alike) : Display
  Divide : Product  Inputs=*/
  Gain : Gain  Gain=-1
  Gain2 : Gain  Gain=-1
  Kd : Constant  Value=0
  Ki : Gain  Gain=0.1
  Logical Operator : Logic  Operator=OR  AllPortsSameDT=off  OutDataTypeStr=boolean
  PID Controller : slpidlib/PID Controller  Controller=P  Form=Parallel  TimeDomain=Continuous-time  UseExternalTs=off  SampleTime=-1  IntegratorMethod=Forward Euler  FilterMethod=Forward Euler  ControllerParametersSource=internal  P=0.5  I=1  UseKiTs=off  D=0  UseExternalDerivativeSource=off  N=100  UseFilter=on  TunerSelectOption=Transfer Function Based (PID Tuner App)  InitialConditionSource=internal  InitialConditionForIntegrator=0  InitialConditionForFilter=0  DifferentiatorICPrevScaledInput=0  ExternalReset=none  TrackingMode=off  Kt=1  LimitOutput=off  SatLimitsSource=internal  UpperSaturationLimit=inf  LowerSaturationLimit=-inf  LinearizeAsGain=on  AntiWindupMode=none  Kb=1  LimitIntegrator=off  UpperIntegratorSaturationLimit=inf  LowerIntegratorSaturationLimit=-inf  POutMin=[]  POutMax=[]  IOutMin=[]  IOutMax=[]  DOutMin=[]  DOutMax=[]  NOutMin=[]  NOutMax=[]  SumOutMin=[]  SumOutMax=[]  SaturationOutMin=[]  SaturationOutMax=[]  PParamMin=[]  PParamMax=[]  IParamMin=[]  IParamMax=[]  DParamMin=[]  DParamMax=[]  NParamMin=[]  NParamMax=[]  KbParamMin=[]  KbParamMax=[]  KtParamMin=[]  KtParamMax=[]  KbOutMin=[]  KbOutMax=[]  KtOutMin=[]  KtOutMax=[]  IntegratorOutMin=[]  IntegratorOutMax=[]  FilterOutMin=[]  FilterOutMax=[]  SumI1OutMin=[]  SumI1OutMax=[]  SumI2OutMin=[]  SumI2OutMax=[]  SumI3OutMin=[]  SumI3OutMax=[]  SumI4OutMin=[]  SumI4OutMax=[]  SumDOutMin=[]  SumDOutMax=[]  DifferentiatorOutMin=[]  DifferentiatorOutMax=[]  FilterDiffOutCoefMin=[]  FilterDiffOutCoefMax=[]  ReciprocalOutMin=[]  ReciprocalOutMax=[]  SumDenOutMin=[]  SumDenOutMax=[]  SumNumOutMin=[]  SumNumOutMax=[]  DivideOutMin=[]  DivideOutMax=[]  UdiffTsProdOutMin=[]  UdiffTsProdOutMax=[]  NTsProdOutMin=[]  NTsProdOutMax=[]  UintegralTsProdOutMin=[]  UintegralTsProdOutMax=[]  UngainTsProdOutMin=[]  UngainTsProdOutMax=[]  ClampingZeroOutDataTypeStr=Inherit: Inherit via back propagation  ClampingZeroOutMin=[]  ClampingZeroOutMax=[]  FilterDenConstantOutDataTypeStr=Inherit: Inherit via back propagation  FilterDenConstantOutMin=[]  FilterDenConstantOutMax=[]  PCopyOutDataTypeStr=Inherit: Inherit via back propagation  PCopyOutMin=[]  PCopyOutMax=[]  NCopyOutDataTypeStr=Inherit: Inherit via back propagation  NCopyOutMin=[]  NCopyOutMax=[]  IntegratorContinuousStateAttributes=''  IntegratorStateMustResolveToSignalObject=off  IntegratorRTWStateStorageClass=Auto  FilterContinuousStateAttributes=''  FilterStateMustResolveToSignalObject=off  FilterRTWStateStorageClass=Auto  ParallelPVariant=InternalParameters  IdealPVariant=Disabled  IVariant=Disabled  DVariant=Disabled  IntegratorVariant=Disabled  SatVariant=Disabled  AWVariant=Disabled  PCopyVariant=Disabled  TRVariant=Disabled  FdbkBlocksVariant=Forward  IdealPFdbkVariant=Disabled  SatFdbkVariant=Disabled  DerivativeFilterVariant=Disabled  NVariant=Disabled  NCopyVariant=Disabled_SignalSpec  FilterICVariant=Disabled  IntegratorICVariant=Disabled  ExternalResetVariant=Disabled  TRSumVariant=Passthrough  SumFdbkVariant=Disabled  SumVariant=Passthrough_P  TsampFilterVariant=InternalTs  TsampNgainVariant=Passthrough  TsampIntegralVariant=Disabled_SignalSpec  ExternalSaturationOutDataTypeStr=Inherit: Same as second input  DerivativeSourceVariant=Disabled  PreIntVariant=InternalPreInt
  PID Controller1 : slpidlib/PID Controller  Controller=P  Form=Parallel  TimeDomain=Continuous-time  UseExternalTs=off  SampleTime=-1  IntegratorMethod=Forward Euler  FilterMethod=Forward Euler  ControllerParametersSource=internal  P=1  I=1  UseKiTs=off  D=0  UseExternalDerivativeSource=off  N=100  UseFilter=on  TunerSelectOption=Transfer Function Based (PID Tuner App)  InitialConditionSource=internal  InitialConditionForIntegrator=0  InitialConditionForFilter=0  DifferentiatorICPrevScaledInput=0  ExternalReset=none  TrackingMode=off  Kt=1  LimitOutput=off  SatLimitsSource=internal  UpperSaturationLimit=inf  LowerSaturationLimit=-inf  LinearizeAsGain=on  AntiWindupMode=none  Kb=1  LimitIntegrator=off  UpperIntegratorSaturationLimit=inf  LowerIntegratorSaturationLimit=-inf  POutMin=[]  POutMax=[]  IOutMin=[]  IOutMax=[]  DOutMin=[]  DOutMax=[]  NOutMin=[]  NOutMax=[]  SumOutMin=[]  SumOutMax=[]  SaturationOutMin=[]  SaturationOutMax=[]  PParamMin=[]  PParamMax=[]  IParamMin=[]  IParamMax=[]  DParamMin=[]  DParamMax=[]  NParamMin=[]  NParamMax=[]  KbParamMin=[]  KbParamMax=[]  KtParamMin=[]  KtParamMax=[]  KbOutMin=[]  KbOutMax=[]  KtOutMin=[]  KtOutMax=[]  IntegratorOutMin=[]  IntegratorOutMax=[]  FilterOutMin=[]  FilterOutMax=[]  SumI1OutMin=[]  SumI1OutMax=[]  SumI2OutMin=[]  SumI2OutMax=[]  SumI3OutMin=[]  SumI3OutMax=[]  SumI4OutMin=[]  SumI4OutMax=[]  SumDOutMin=[]  SumDOutMax=[]  DifferentiatorOutMin=[]  DifferentiatorOutMax=[]  FilterDiffOutCoefMin=[]  FilterDiffOutCoefMax=[]  ReciprocalOutMin=[]  ReciprocalOutMax=[]  SumDenOutMin=[]  SumDenOutMax=[]  SumNumOutMin=[]  SumNumOutMax=[]  DivideOutMin=[]  DivideOutMax=[]  UdiffTsProdOutMin=[]  UdiffTsProdOutMax=[]  NTsProdOutMin=[]  NTsProdOutMax=[]  UintegralTsProdOutMin=[]  UintegralTsProdOutMax=[]  UngainTsProdOutMin=[]  UngainTsProdOutMax=[]  ClampingZeroOutDataTypeStr=Inherit: Inherit via back propagation  ClampingZeroOutMin=[]  ClampingZeroOutMax=[]  FilterDenConstantOutDataTypeStr=Inherit: Inherit via back propagation  FilterDenConstantOutMin=[]  FilterDenConstantOutMax=[]  PCopyOutDataTypeStr=Inherit: Inherit via back propagation  PCopyOutMin=[]  PCopyOutMax=[]  NCopyOutDataTypeStr=Inherit: Inherit via back propagation  NCopyOutMin=[]  NCopyOutMax=[]  IntegratorContinuousStateAttributes=''  IntegratorStateMustResolveToSignalObject=off  IntegratorRTWStateStorageClass=Auto  FilterContinuousStateAttributes=''  FilterStateMustResolveToSignalObject=off  FilterRTWStateStorageClass=Auto  ParallelPVariant=InternalParameters  IdealPVariant=Disabled  IVariant=Disabled  DVariant=Disabled  IntegratorVariant=Disabled  SatVariant=Disabled  AWVariant=Disabled  PCopyVariant=Disabled  TRVariant=Disabled  FdbkBlocksVariant=Forward  IdealPFdbkVariant=Disabled  SatFdbkVariant=Disabled  DerivativeFilterVariant=Disabled  NVariant=Disabled  NCopyVariant=Disabled_SignalSpec  FilterICVariant=Disabled  IntegratorICVariant=Disabled  ExternalResetVariant=Disabled  TRSumVariant=Passthrough  SumFdbkVariant=Disabled  SumVariant=Passthrough_P  TsampFilterVariant=InternalTs  TsampNgainVariant=Passthrough  TsampIntegralVariant=Disabled_SignalSpec  ExternalSaturationOutDataTypeStr=Inherit: Same as second input  DerivativeSourceVariant=Disabled  PreIntVariant=InternalPreInt
  Product{,1..4} (5 alike) : Product
  Relational Operator : RelationalOperator  OutDataTypeStr=boolean  RndMeth=Simplest  InputSameDT=off
  Relational Operator1 : RelationalOperator  Operator=<=  OutDataTypeStr=boolean  RndMeth=Simplest  InputSameDT=off
  Relational Operator2 : RelationalOperator  Operator=>  OutDataTypeStr=boolean  RndMeth=Simplest  InputSameDT=off
  Relational Operator3 : RelationalOperator  Operator=<  OutDataTypeStr=boolean  RndMeth=Simplest  InputSameDT=off
  Saturation1 : Saturate  LowerLimit=-0.7
  Saturation2 : Saturate  UpperLimit=0.3  LowerLimit=-0.2
  Saturation3 : Saturate  UpperLimit=0.7  LowerLimit=0
  Saturation4 : Saturate  UpperLimit=1  LowerLimit=0.7
  Selector : Selector  InputPortWidth=3  IndexOptions=Index vector (dialog)  Indices=[3]  OutputSizes=1
  Selector1 : Selector  InputPortWidth=3  IndexOptions=Index vector (dialog)  Indices=[3]  OutputSizes=1
  Selector2 : Selector  InputPortWidth=3  IndexOptions=Index vector (dialog)  Indices=[3]  OutputSizes=1
  Sum{,1,3..4} (4 alike) : Sum  Inputs=|+-
  Sum5 : Sum  Inputs=|++
  Sum6 : Sum  Inputs=|++
  Sum7 : Sum  Inputs=|++
  Switch : Switch  Criteria=u2 > Threshold  SaturateOnIntegerOverflow=off  InputSameDT=off
  Switch1 : Switch  Criteria=u2 > Threshold  SaturateOnIntegerOverflow=off  InputSameDT=off
  Terminator : Terminator
  Trigonometric Function : Trigonometry  Operator=cos
  Trigonometric Function1 : Trigonometry  Operator=cos
  Unary Minus : UnaryMinus
  Unit Delay2 : UnitDelay  SampleTime=-1  HasFrameUpgradeWarning=on
  block_down : Logic  AllPortsSameDT=off  OutDataTypeStr=boolean
  block_up : Logic  AllPortsSameDT=off  OutDataTypeStr=boolean
  dt : Constant  Value=0.005
  commanded thrust : Outport
  wires:
  Selector/1 -> Gain/1
  Bus Selector/1 -> Selector/1  "<Xe>"
  Bus Selector/2 -> Selector1/1  "<Ve>"
  Altitude controller/1 -> Saturation1/1
  Sum/1 -> Altitude controller/1
  Gain/1 -> Sum/2, Display/1
  Ref Alt/1 -> Gain2/1
  Gain2/1 -> Display4/1, Sum/1
  Sum4/1 -> Product/2, [e_v]  "e_v"
  Sum3/1 -> Switch1/1
  Relational Operator/1 -> block_up/1  "sag_hi"
  Constant/1 -> Sum3/2, Sum6/2
  [delta_i] -> Sum5/2
  Saturation3/1 -> Relational Operator/1, Display2/1, commanded thrust/1, Relational Operator1/1
  Relational Operator2/1 -> block_up/2  "dI_pos"
  Switch/1 -> Display10/1, [delta_i]
  Detect Rise Positive1/1 -> Switch1/2
  Constant7/1 -> Switch/1
  Unit Delay2/1 -> Sum5/1, Sum6/1
  Bus Selector1/1 -> Demux/1  "<Euler>"
  throttlecmd/1 -> Display3/1, Sum3/1
  Relational Operator3/1 -> block_down/2  "dI_neg"
  States/1 -> Bus Selector1/1, Bus Selector/1
  Demux/3 -> Terminator/1
  Sum5/1 -> Saturation2/1
  Constant6/1 -> Relational Operator3/2
  Saturation1/1 -> Display1/1, Sum4/1
  block_up/1 -> Logical Operator/1
  Product2/1 -> Saturation3/1
  Constant4/1 -> Relational Operator1/2
  Saturation2/1 -> Display6/1, Switch1/3
  Trigonometric Function1/1 -> Product1/2
  Constant5/1 -> Relational Operator2/2
  Switch1/1 -> Display7/1, Unit Delay2/1
  Demux/2 -> Trigonometric Function1/1
  Relational Operator1/1 -> block_down/1  "sag_lo"
  Constant3/1 -> Relational Operator/2
  Demux/1 -> Trigonometric Function/1
  Divide/1 -> Product2/2  "tilt_comp"
  Saturation4/1 -> Divide/2  "cos_tilt_limited"
  Product/1 -> Ki/1
  Logical Operator/1 -> Switch/2
  block_down/1 -> Logical Operator/2
  Constant2/1 -> Divide/1
  Product1/1 -> Saturation4/1
  Trigonometric Function/1 -> Product1/1
  Unary Minus/1 -> Sum4/2
  trigger/1 -> Display5/1, Detect Rise Positive1/1
  Sum6/1 -> Sum7/1
  Sum7/1 -> Display8/1, Product2/1
  [e_v] -> PID Controller/1
  PID Controller/1 -> Sum7/2
  Selector1/1 -> Unary Minus/1
  Ki/1 -> Display9/1, Switch/3, Relational Operator2/1, Relational Operator3/1
  dt/1 -> Product/1
  [e_v] -> PID Controller1/1
  [e_v] -> Product3/2
  Bus Selector/3 -> Selector2/1  "<Abb>"
  Selector2/1 -> Product4/2
  Kd/1 -> Product4/1
  Product4/1 -> Sum1/2  "Kd*vel_dot_z"
  Product3/1 -> Discrete-Time Integrator/1  "Ki*vel_error_z"
  Constant1/1 -> Product3/1
  Discrete-Time Integrator/1 -> Sum1/1
